simulink model "solar_grid_powered_EV_Battery_Charging_station"  (R2020a)
settings: Solver=VariableStepAuto  StartTime=0.0  StopTime=1  RelTol=1e-3
undefined symbols (not defined in the file): Ion, Lithium
libraries: powerlib x68, simulink x10, powerlib_meascontrol x4, electricdrivelib x1, re_lib x1
(part 2 of 2)

== system solar_grid_powered_EV_Battery_Charging_station/Controller & Converter/Bidirectional converter with battery controller/controller/Duty Cycle ==
  Vb : Inport
  PID Controller1 : simulink/Continuous/PID Controller  Controller=PID  Form=Parallel  TimeDomain=Continuous-time  UseExternalTs=off  SampleTime=-1  IntegratorMethod=Forward Euler  FilterMethod=Forward Euler  ControllerParametersSource=internal  P=.02  I=0  D=0  UseFilter=on  N=100  TunerSelectOption=Transfer Function Based (PID Tuner App)  InitialConditionSource=internal  InitialConditionForIntegrator=0  InitialConditionForFilter=0  DifferentiatorICPrevScaledInput=0  ExternalReset=none  TrackingMode=off  Kt=1  LimitOutput=off  UpperSaturationLimit=inf  LowerSaturationLimit=-inf  LinearizeAsGain=on  AntiWindupMode=none  Kb=1  POutMin=[]  POutMax=[]  IOutMin=[]  IOutMax=[]  DOutMin=[]  DOutMax=[]  NOutMin=[]  NOutMax=[]  SumOutMin=[]  SumOutMax=[]  SaturationOutMin=[]  SaturationOutMax=[]  PParamMin=[]  PParamMax=[]  IParamMin=[]  IParamMax=[]  DParamMin=[]  DParamMax=[]  NParamMin=[]  NParamMax=[]  KbParamMin=[]  KbParamMax=[]  KtParamMin=[]  KtParamMax=[]  KbOutMin=[]  KbOutMax=[]  KtOutMin=[]  KtOutMax=[]  IntegratorOutMin=[]  IntegratorOutMax=[]  FilterOutMin=[]  FilterOutMax=[]  SumI1OutMin=[]  SumI1OutMax=[]  SumI2OutMin=[]  SumI2OutMax=[]  SumI3OutMin=[]  SumI3OutMax=[]  SumI4OutMin=[]  SumI4OutMax=[]  SumDOutMin=[]  SumDOutMax=[]  DifferentiatorOutMin=[]  DifferentiatorOutMax=[]  FilterDiffOutCoefMin=[]  FilterDiffOutCoefMax=[]  ReciprocalOutMin=[]  ReciprocalOutMax=[]  SumDenOutMin=[]  SumDenOutMax=[]  SumNumOutMin=[]  SumNumOutMax=[]  DivideOutMin=[]  DivideOutMax=[]  UdiffTsProdOutMin=[]  UdiffTsProdOutMax=[]  NTsProdOutMin=[]  NTsProdOutMax=[]  UintegralTsProdOutMin=[]  UintegralTsProdOutMax=[]  UngainTsProdOutMin=[]  UngainTsProdOutMax=[]  IntegratorContinuousStateAttributes=''  IntegratorStateMustResolveToSignalObject=off  IntegratorRTWStateStorageClass=Auto  FilterContinuousStateAttributes=''  FilterStateMustResolveToSignalObject=off  FilterRTWStateStorageClass=Auto  ParallelPVariant=InternalParameters  IdealPVariant=Disabled  IVariant=InternalParameters  DVariant=InternalParameters  IntegratorVariant=Continuous  SatVariant=Disabled  AWVariant=Passthrough  PCopyVariant=Disabled  TRVariant=Disabled  FdbkBlocksVariant=Forward  IdealPFdbkVariant=Disabled  SatFdbkVariant=Disabled  DerivativeFilterVariant=ContFilter  NVariant=InternalParameters  NCopyVariant=Disabled  FilterICVariant=InternalICsFilter  IntegratorICVariant=InternalICs  ExternalResetVariant=Disabled  TRSumVariant=Passthrough  SumFdbkVariant=Disabled  SumVariant=Sum_PID  TsampFilterVariant=InternalTs  TsampNgainVariant=Passthrough  TsampIntegralVariant=Passthrough
  Sum : Sum  Inputs=|+-
  Vb* : Constant  Value=290
  D : Outport
  wires:
  Vb*/1 -> Sum/1
  Vb/1 -> Sum/2
  Sum/1 -> PID Controller1/1
  PID Controller1/1 -> D/1

== system solar_grid_powered_EV_Battery_Charging_station/Controller & Converter/Bidirectional converter with battery controller/controller/Duty Cycle1 ==
  Vin : Inport
  Ib : Inport  Port=2
  PID Controller1 : simulink/Continuous/PID Controller  Controller=PID  Form=Parallel  TimeDomain=Continuous-time  UseExternalTs=off  SampleTime=-1  IntegratorMethod=Forward Euler  FilterMethod=Forward Euler  ControllerParametersSource=internal  P=.1  I=0  D=0  UseFilter=on  N=100  TunerSelectOption=Transfer Function Based (PID Tuner App)  InitialConditionSource=internal  InitialConditionForIntegrator=0  InitialConditionForFilter=0  DifferentiatorICPrevScaledInput=0  ExternalReset=none  TrackingMode=off  Kt=1  LimitOutput=off  UpperSaturationLimit=inf  LowerSaturationLimit=-inf  LinearizeAsGain=on  AntiWindupMode=none  Kb=1  POutMin=[]  POutMax=[]  IOutMin=[]  IOutMax=[]  DOutMin=[]  DOutMax=[]  NOutMin=[]  NOutMax=[]  SumOutMin=[]  SumOutMax=[]  SaturationOutMin=[]  SaturationOutMax=[]  PParamMin=[]  PParamMax=[]  IParamMin=[]  IParamMax=[]  DParamMin=[]  DParamMax=[]  NParamMin=[]  NParamMax=[]  KbParamMin=[]  KbParamMax=[]  KtParamMin=[]  KtParamMax=[]  KbOutMin=[]  KbOutMax=[]  KtOutMin=[]  KtOutMax=[]  IntegratorOutMin=[]  IntegratorOutMax=[]  FilterOutMin=[]  FilterOutMax=[]  SumI1OutMin=[]  SumI1OutMax=[]  SumI2OutMin=[]  SumI2OutMax=[]  SumI3OutMin=[]  SumI3OutMax=[]  SumI4OutMin=[]  SumI4OutMax=[]  SumDOutMin=[]  SumDOutMax=[]  DifferentiatorOutMin=[]  DifferentiatorOutMax=[]  FilterDiffOutCoefMin=[]  FilterDiffOutCoefMax=[]  ReciprocalOutMin=[]  ReciprocalOutMax=[]  SumDenOutMin=[]  SumDenOutMax=[]  SumNumOutMin=[]  SumNumOutMax=[]  DivideOutMin=[]  DivideOutMax=[]  UdiffTsProdOutMin=[]  UdiffTsProdOutMax=[]  NTsProdOutMin=[]  NTsProdOutMax=[]  UintegralTsProdOutMin=[]  UintegralTsProdOutMax=[]  UngainTsProdOutMin=[]  UngainTsProdOutMax=[]  IntegratorContinuousStateAttributes=''  IntegratorStateMustResolveToSignalObject=off  IntegratorRTWStateStorageClass=Auto  FilterContinuousStateAttributes=''  FilterStateMustResolveToSignalObject=off  FilterRTWStateStorageClass=Auto  ParallelPVariant=InternalParameters  IdealPVariant=Disabled  IVariant=InternalParameters  DVariant=InternalParameters  IntegratorVariant=Continuous  SatVariant=Disabled  AWVariant=Passthrough  PCopyVariant=Disabled  TRVariant=Disabled  FdbkBlocksVariant=Forward  IdealPFdbkVariant=Disabled  SatFdbkVariant=Disabled  DerivativeFilterVariant=ContFilter  NVariant=InternalParameters  NCopyVariant=Disabled  FilterICVariant=InternalICsFilter  IntegratorICVariant=InternalICs  ExternalResetVariant=Disabled  TRSumVariant=Passthrough  SumFdbkVariant=Disabled  SumVariant=Sum_PID  TsampFilterVariant=InternalTs  TsampNgainVariant=Passthrough  TsampIntegralVariant=Passthrough
  PID Controller2 : simulink/Continuous/PID Controller  Controller=PID  Form=Parallel  TimeDomain=Continuous-time  UseExternalTs=off  SampleTime=-1  IntegratorMethod=Forward Euler  FilterMethod=Forward Euler  ControllerParametersSource=internal  P=1  I=0  D=0  UseFilter=on  N=100  TunerSelectOption=Transfer Function Based (PID Tuner App)  InitialConditionSource=internal  InitialConditionForIntegrator=0  InitialConditionForFilter=0  DifferentiatorICPrevScaledInput=0  ExternalReset=none  TrackingMode=off  Kt=1  LimitOutput=off  UpperSaturationLimit=inf  LowerSaturationLimit=-inf  LinearizeAsGain=on  AntiWindupMode=none  Kb=1  POutMin=[]  POutMax=[]  IOutMin=[]  IOutMax=[]  DOutMin=[]  DOutMax=[]  NOutMin=[]  NOutMax=[]  SumOutMin=[]  SumOutMax=[]  SaturationOutMin=[]  SaturationOutMax=[]  PParamMin=[]  PParamMax=[]  IParamMin=[]  IParamMax=[]  DParamMin=[]  DParamMax=[]  NParamMin=[]  NParamMax=[]  KbParamMin=[]  KbParamMax=[]  KtParamMin=[]  KtParamMax=[]  KbOutMin=[]  KbOutMax=[]  KtOutMin=[]  KtOutMax=[]  IntegratorOutMin=[]  IntegratorOutMax=[]  FilterOutMin=[]  FilterOutMax=[]  SumI1OutMin=[]  SumI1OutMax=[]  SumI2OutMin=[]  SumI2OutMax=[]  SumI3OutMin=[]  SumI3OutMax=[]  SumI4OutMin=[]  SumI4OutMax=[]  SumDOutMin=[]  SumDOutMax=[]  DifferentiatorOutMin=[]  DifferentiatorOutMax=[]  FilterDiffOutCoefMin=[]  FilterDiffOutCoefMax=[]  ReciprocalOutMin=[]  ReciprocalOutMax=[]  SumDenOutMin=[]  SumDenOutMax=[]  SumNumOutMin=[]  SumNumOutMax=[]  DivideOutMin=[]  DivideOutMax=[]  UdiffTsProdOutMin=[]  UdiffTsProdOutMax=[]  NTsProdOutMin=[]  NTsProdOutMax=[]  UintegralTsProdOutMin=[]  UintegralTsProdOutMax=[]  UngainTsProdOutMin=[]  UngainTsProdOutMax=[]  IntegratorContinuousStateAttributes=''  IntegratorStateMustResolveToSignalObject=off  IntegratorRTWStateStorageClass=Auto  FilterContinuousStateAttributes=''  FilterStateMustResolveToSignalObject=off  FilterRTWStateStorageClass=Auto  ParallelPVariant=InternalParameters  IdealPVariant=Disabled  IVariant=InternalParameters  DVariant=InternalParameters  IntegratorVariant=Continuous  SatVariant=Disabled  AWVariant=Passthrough  PCopyVariant=Disabled  TRVariant=Disabled  FdbkBlocksVariant=Forward  IdealPFdbkVariant=Disabled  SatFdbkVariant=Disabled  DerivativeFilterVariant=ContFilter  NVariant=InternalParameters  NCopyVariant=Disabled  FilterICVariant=InternalICsFilter  IntegratorICVariant=InternalICs  ExternalResetVariant=Disabled  TRSumVariant=Passthrough  SumFdbkVariant=Disabled  SumVariant=Sum_PID  TsampFilterVariant=InternalTs  TsampNgainVariant=Passthrough  TsampIntegralVariant=Passthrough
  Sum : Sum  Inputs=|+-
  Sum1 : Sum  Inputs=|++
  Vb* : Constant  Value=698
  D : Outport
  wires:
  Vb*/1 -> Sum/1
  Vin/1 -> Sum/2
  Sum/1 -> PID Controller1/1
  Ib/1 -> Sum1/2
  Sum1/1 -> PID Controller2/1
  PID Controller1/1 -> Sum1/1
  PID Controller2/1 -> D/1

== system solar_grid_powered_EV_Battery_Charging_station/Controller & Converter/Bidirectional converter with battery controller/controller/pwm ==
  Duty : Inport
  Relational Operator : RelationalOperator  OutDataTypeStr=boolean  RndMeth=Nearest
  Repeating Sequence : simulink/Sources/Repeating Sequence  rep_seq_t=[0 1/10000]  rep_seq_y=[0 1]
  Scope : Scope
  Scope1 : Scope
  pwm : Outport
  wires:
  Repeating Sequence/1 -> Relational Operator/2, Scope/1
  Relational Operator/1 -> Scope1/1, pwm/1
  Duty/1 -> Relational Operator/1

== system solar_grid_powered_EV_Battery_Charging_station/Controller & Converter/Bidirectional converter with battery controller/controller/pwm1 ==
  Duty : Inport
  Relational Operator : RelationalOperator  OutDataTypeStr=boolean  RndMeth=Nearest
  Repeating Sequence : simulink/Sources/Repeating Sequence  rep_seq_t=[0 1/10000]  rep_seq_y=[0 1]
  Scope : Scope
  Scope1 : Scope
  pwm : Outport
  wires:
  Repeating Sequence/1 -> Relational Operator/2, Scope/1
  Relational Operator/1 -> Scope1/1, pwm/1
  Duty/1 -> Relational Operator/1

== system solar_grid_powered_EV_Battery_Charging_station/Controller & Converter/AC-DC & DC-AC Converter/controller1/MSOGI_FLL1/FLL ==
  note: ώ
  v’ : Inport
  qv’ : Inport  Port=2
  ξ : Inport  Port=3
  Constant : Constant  Value=2*3.14*50
  Divide : Product  Inputs=*/
  Divide1 : Product  Inputs=**
  Divide2 : Product  Inputs=**
  Divide3 : Product  Inputs=**
  Integrator : Integrator
  Kl : Gain  Gain=1.28
  Sum : Sum
  Sum1 : Sum  Inputs=|++
  ϒ : Gain  Gain=-0.26
  ώ : Outport
  wires:
  ϒ/1 -> Divide3/1
  v’/1 -> Divide2/2, Divide2/1
  Divide2/1 -> Sum/1
  Constant/1 -> Sum1/1
  Divide/1 -> Divide3/2
  Sum1/1 -> Kl/1, ώ/1
  Divide3/1 -> Integrator/1
  ξ/1 -> ϒ/1
  qv’/1 -> Divide1/1, Divide1/2
  Sum/1 -> Divide/1
  Integrator/1 -> Sum1/2
  Kl/1 -> Divide/2
  Divide1/1 -> Sum/2

== system solar_grid_powered_EV_Battery_Charging_station/Controller & Converter/AC-DC & DC-AC Converter/controller1/MSOGI_FLL1/MSOGI ==
  V : Inport
  ώ : Inport  Port=2
  MSOGI : Subsystem
  V'α : Outport
  qv'α : Outport  Port=2
  ξ : Outport  Port=3
  wires:
  V/1 -> MSOGI/1(V)
  MSOGI/1(v’α) -> V'α/1
  MSOGI/2(qv’α) -> qv'α/1
  ώ/1 -> MSOGI/2(ώ)
  MSOGI/3(ξ) -> ξ/1

== system solar_grid_powered_EV_Battery_Charging_station/Controller & Converter/AC-DC & DC-AC Converter/controller1/MSOGI_FLL1/MSOGI1 ==
  ώ : Inport
  V : Inport  Port=2
  MSOGI : Subsystem
  V'β : Outport
  qv'β : Outport  Port=2
  wires:
  V/1 -> MSOGI/1(V)
  MSOGI/1(v’β) -> V'β/1
  MSOGI/2(qv’β) -> qv'β/1
  ώ/1 -> MSOGI/2(ώ)

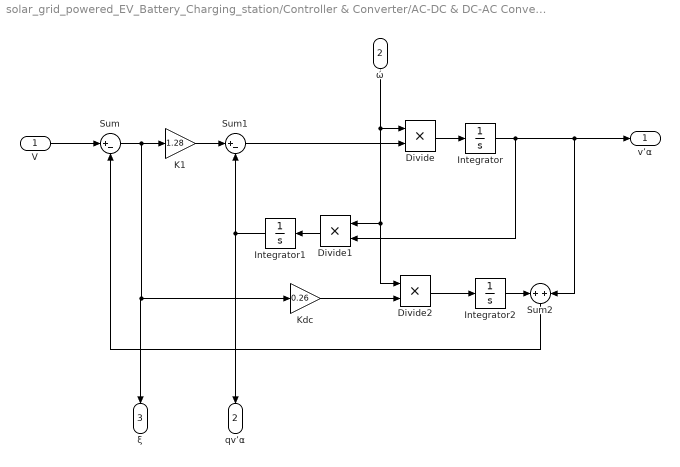
== system solar_grid_powered_EV_Battery_Charging_station/Controller & Converter/AC-DC & DC-AC Converter/controller1/MSOGI_FLL1/MSOGI/MSOGI ==
  V : Inport
  ώ : Inport  Port=2
  Divide : Product  Inputs=**
  Divide1 : Product  Inputs=**
  Divide2 : Product  Inputs=**
  Integrator : Integrator
  Integrator1 : Integrator
  Integrator2 : Integrator
  K1 : Gain  Gain=1.28
  Kdc : Gain  Gain=0.26
  Sum : Sum  Inputs=|+-
  Sum1 : Sum  Inputs=|+-
  Sum2 : Sum
  v’α : Outport
  qv’α : Outport  Port=2
  ξ : Outport  Port=3
  wires:
  Integrator1/1 -> qv’α/1, Sum1/2
  Divide1/1 -> Integrator1/1
  ώ/1 -> Divide2/1, Divide1/1, Divide/1
  Integrator2/1 -> Sum2/1
  Integrator/1 -> Divide1/2, v’α/1, Sum2/2
  Sum/1 -> K1/1, ξ/1, Kdc/1
  Kdc/1 -> Divide2/2
  Sum2/1 -> Sum/2
  V/1 -> Sum/1
  Sum1/1 -> Divide/2
  K1/1 -> Sum1/1
  Divide2/1 -> Integrator2/1
  Divide/1 -> Integrator/1

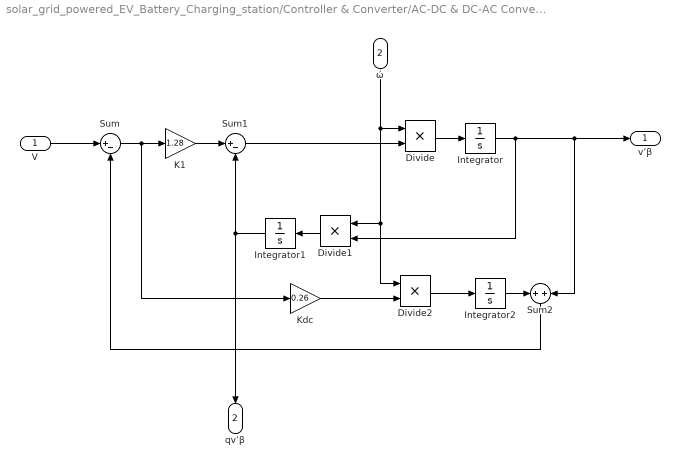
== system solar_grid_powered_EV_Battery_Charging_station/Controller & Converter/AC-DC & DC-AC Converter/controller1/MSOGI_FLL1/MSOGI1/MSOGI ==
  V : Inport
  ώ : Inport  Port=2
  Divide : Product  Inputs=**
  Divide1 : Product  Inputs=**
  Divide2 : Product  Inputs=**
  Integrator : Integrator
  Integrator1 : Integrator
  Integrator2 : Integrator
  K1 : Gain  Gain=1.28
  Kdc : Gain  Gain=0.26
  Sum : Sum  Inputs=|+-
  Sum1 : Sum  Inputs=|+-
  Sum2 : Sum
  v’β : Outport
  qv’β : Outport  Port=2
  wires:
  Integrator1/1 -> qv’β/1, Sum1/2
  Divide1/1 -> Integrator1/1
  ώ/1 -> Divide2/1, Divide1/1, Divide/1
  Integrator2/1 -> Sum2/1
  Integrator/1 -> Divide1/2, v’β/1, Sum2/2
  Sum/1 -> K1/1, Kdc/1
  Kdc/1 -> Divide2/2
  Sum2/1 -> Sum/2
  V/1 -> Sum/1
  Sum1/1 -> Divide/2
  K1/1 -> Sum1/1
  Divide2/1 -> Integrator2/1
  Divide/1 -> Integrator/1

== matlab function solar_grid_powered_EV_Battery_Charging_station/Controller & Converter/MPPT/P&O_MPPT ==
  data: Vpv input; D output; Ipv input
function D = P_and_O(Vpv,Ipv)

% initilization
Dmax = 0.95;
Dmin = 0;
Dinit = 0.95;
deltaD = 0.001;

persistent Dprev Pprev Vprev

dataType = 'double';

if isempty(Vprev)
    Dprev =.8;
    Vprev = 280;
    Pprev =Dinit;
end


%calculate measured array power
Ppv= Vpv*Ipv;
dv = Vpv-Vprev;
dp = Ppv-Pprev;
%increase or decrease duty cycle based on conditiond

if dp ~=0
    if dp<0
        if dv<0
            D=Dprev-deltaD;
        else
            D=Dprev+deltaD;
        end
    else
        if dv<0
            D=Dprev+deltaD;
        else
            D=Dprev-deltaD;
        end
    end
else
    D=Dprev;
end
if D>=Dmax||D<=Dmin
    D=Dprev;
end
   
% update internal values
Dprev= D;
Vprev =Vpv;
Pprev = Ppv;
